simulink model "dinamicaralik"  (R2023b)
settings: Solver=ode45  StartTime=0.0  StopTime=50  FixedStep=0.0001  RelTol=1e-3
InitFcn:
  | Kpz = 0.3 ;
  | KIz = 0;
  | 
  | bh = 0.010290;  % batan hacim m^3
  | m = 10.5     ;  % aracın kütlesi kg
  | g = 9.81     ;  % yer çekimi ivmesi
  | p = 1000     ; % kg / m^3 yogunluk
  | W = m*g      ;  % aracın agırlıgı N
  | B = p*g*bh   ;  % Kaldırma kuvveti  N
  | 
  | xg = 0 ; % rgid body frame e göre ağırlık merkzi kordinatları
  | yg = 0 ;
  | zg = 0.02 ;
  | 
  | Ix = 0.1011 ; % kg *  m ^2
  | Iy = 0.1159 ;
  | Iz = 0.1615 ;
  | 
  | thrustCoefficient = 50/21.5 ;
  | 
  | % Add mass parametreleri
  | Xu_dot = -5.5;   % Surge direction
  | Yv_dot = -12.7;  % Sway direction
  | Zw_dot = -14.57; % Heave direction
  | 
  | Kp_dot = -0.12;  % Roll moment
  | Mq_dot = -0.12;  % Pitch moment
  | Nr_dot = -0.12;  % Yaw moment
  | 
  | % Linear Damping Values (Doğrusal Sönümleme Katsayıları)
  | Xu = -4.03;   % Ns/m
  | Yv = -6.22;   % Ns/m
  | Zw = -5.18;   % Ns/m
  | Kp = -0.07;   % Ns/rad
  | Mq = -0.07;   % Ns/rad
  | Nr = -0.07;   % Ns/rad
  | 
  | % Quadratic Damping Values (Doğrusal Olmayan Sönümleme Katsayıları)
  | Xuu = -18.18;  % Ns^2/m^2
  | Yvv = -21.66;  % Ns^2/m^2
  | Zww = -36.99;  % Ns^2/m^2
  | Kpp = -1.55;   % Ns^2/rad^2
  | Mqq = -1.55;   % Ns^2/rad^2
  | Nrr = -1.55;   % Ns^2/rad^2
undefined symbols (not defined in the file or in its folder): smiData, X, Y, Z
libraries: slpidlib x41, nesl_utility x14, sm_lib x12
(part 7 of 7)

== matlab function dinamicaralik/Subsystem3/CRB/MATLAB Function ==
  data: V input; y output
function y = fcn(V)

u = V(1);
v = V(2);
w = V(3);

p = V(4);
q = V(5);
r = V(6);

Ix = 0.1011 ; % kg *  m ^2 
Iy = 0.1159 ;
Iz = 0.1615 ;

m = 10.5     ;  % aracın kütlesi kg

% Matrisin tanımlanması
CRB = [
        0,     0,     0,        0,   m*w,    0;
        0,     0,     0,     -m*w,     0,    0;
        0,     0,     0,      m*v,  -m*u,    0;
        0,     m*w,  -m*v,    0,     Iz*r,  -Iy*q;
        m*w,  0,    -m*u,   -Iz*r,    0,    Ix*p;
        -m*v,  -m*u,   0,      Iy*q, -Ix*p,   0;
    ];

y= CRB * V ;

== matlab function dinamicaralik/Subsystem3/Damp/MATLAB Function ==
  data: Vw input; y output
function y = fcn(Vw)

u = Vw(1);
v = Vw(2);
w = Vw(3);
p = Vw(4);
q = Vw(5);
r = Vw(6);

% Linear Damping Values (Doğrusal Sönümleme Katsayıları)
Xu = -4.03;   % Ns/m
Yv = -6.22;   % Ns/m
Zw = -5.18;   % Ns/m
Kp = -0.07;   % Ns/rad
Mq = -0.07;   % Ns/rad
Nr = -0.07;   % Ns/rad

% Quadratic Damping Values (Doğrusal Olmayan Sönümleme Katsayıları)
Xuu = -18.18;  % Ns^2/m^2
Yvv = -21.66;  % Ns^2/m^2
Zww = -36.99;  % Ns^2/m^2
Kpp = -1.55;   % Ns^2/rad^2
Mqq = -1.55;   % Ns^2/rad^2
Nrr = -1.55;   % Ns^2/rad^2


D = -[
        Xu + Xuu*abs(u),         0,                 0,                0,                0,                0;
                  0,   Yv + Yvv*abs(v),             0,                0,                0,                0;
                  0,            0,     Zw + Zww*abs(w),             0,                0,                0;
                  0,            0,                 0,   Kp + Kpp*abs(p),             0,                0;
                  0,            0,                 0,                0,   Mq + Mqq*abs(q),             0;
                  0,            0,                 0,                0,                0,   Nr + Nrr*abs(r);
    ];


y = D * Vw ;

== matlab function dinamicaralik/Subsystem3/MA/MATLAB Function ==
  data: accelW input; y output
function y = fcn(accelW)
% Add mass parametreleri
Xu_dot = -5.5;   % Surge direction
Yv_dot = -12.7;  % Sway direction
Zw_dot = -14.57; % Heave direction

Kp_dot = -0.12;  % Roll moment
Mq_dot = -0.12;  % Pitch moment
Nr_dot = -0.12;  % Yaw moment

% MA Matrisinin tanımlanması
MA = -[
        Xu_dot,    0,       0,       0,       0,       0;
        0,       Yv_dot,    0,       0,       0,       0;
        0,         0,     Zw_dot,    0,       0,       0;
        0,         0,       0,     Kp_dot,   0,       0;
        0,         0,       0,       0,     Mq_dot,   0;
        0,         0,       0,       0,       0,     Nr_dot
    ];

y = MA * accelW;

== matlab function dinamicaralik/Subsystem3/inv MA and MRB/MA ve MRB ==
  data: u input; y output
function y = fcn(u)

m = 10.5     ;  % aracın kütlesi kg

xg = 0 ; % rgid body frame e göre ağırlık merkzi kordinatları
yg = 0 ;
zg = 0.02;

Ix = 0.1011 ; % kg *  m ^2 
Iy = 0.1159 ;
Iz = 0.1615 ;


% MRB Matrisinin tanımlanması
MRB = [
        m,    0,    0,    0,   m*zg,  0;
        0,    m,    0, -m*zg,   0,    0;
        0,    0,    m,    0,    0,    0;
        0, -m*zg,   0,   Ix,    0,    0;
       m*zg,  0,    0,    0,   Iy,    0;
        0,    0,    0,    0,    0,   Iz
    ];


Xu_dot = -5.5;   % Surge direction
Yv_dot = -12.7;  % Sway direction
Zw_dot = -14.57; % Heave direction

Kp_dot = -0.12;  % Roll moment
Mq_dot = -0.12;  % Pitch moment
Nr_dot = -0.12;  % Yaw moment

% MA Matrisinin tanımlanması
MA = -[
        Xu_dot,    0,       0,       0,       0,       0;
        0,       Yv_dot,    0,       0,       0,       0;
        0,         0,     Zw_dot,    0,       0,       0;
        0,         0,       0,     Kp_dot,   0,       0;
        0,         0,       0,       0,     Mq_dot,   0;
        0,         0,       0,       0,       0,     Nr_dot
    ];

%inv([m 0 0 0 0 0;0 m 0 0 0 0;0 0 m 0 0 0;0 0 0 Ix 0 0;0 0 0 0 Iy 0;0 0 0 0 0 Iz]+[Xudot 0 0 0 0 0;0 Yvdot 0 0 0 0;0 0 Zwdot 0 0 0;0 0 0 Kpdot 0 0;0 0 0 0 Mqdot 0;0 0 0 0 0 Nrdot])
y = inv(MRB + MA) * u ; % M_product * y = u denkleminden y'i çözer

== matlab function dinamicaralik/Subsystem3/inv MA and MRB/MRB sadece ==
  data: u input; y output
function y = fcn(u)

m = 10.5     ;  % aracın kütlesi kg

xg = 0 ; % rgid body frame e göre ağırlık merkzi kordinatları
yg = 0 ;
zg = 0.02 ;

Ix = 0.1011 ; % kg *  m ^2 
Iy = 0.1159 ;
Iz = 0.1615 ;


% MRB Matrisinin tanımlanması
MRB = [
        m,    0,    0,    0,   m*zg,  0;
        0,    m,    0, -m*zg,   0,    0;
        0,    0,    m,    0,    0,    0;
        0, -m*zg,   0,   Ix,    0,    0;
       m*zg,  0,    0,    0,   Iy,    0;
        0,    0,    0,    0,    0,   Iz
    ];


y = (MRB) \ u ; % M_product * y = u denkleminden y'i çözer

== matlab function dinamicaralik/Subsystem4/MATLAB Function ==
  data: F1 input; thrust1 output
function thrust1 = fcn(F1)

% T1
lx1 = 156 / 1000;  % metre
ly1 = 111 / 1000;  % metre
lz1 = 85 / 1000;   % metre
F1q = pi/4;

Fx = F1 * cos(F1q);
Fy = -F1 * sin(F1q);
Fz = 0;

% Matrisin tanımlanması
forces_and_moments = [
    Fx;                  % Kuvvet: x bileşeni
    Fy;                  % Kuvvet: y bileşeni
    Fz;                  % Kuvvet: z bileşeni
    Fz*ly1 - Fy*lz1;    % Moment: x ekseni etrafında
    Fx*lz1 - Fz*lx1;    % Moment: y ekseni etrafında
    Fy*lx1 - Fx*ly1     % Moment: z ekseni etrafında
];
% Sonuçların görüntülenmesi
%disp('Forces and Moments Matrix:');
%disp(forces_and_moments);

thrust1 = forces_and_moments;

== matlab function dinamicaralik/Subsystem4/MATLAB Function1 ==
  data: F2 input; thrust2 output
function thrust2 = fcn(F2)

% T2
lx2 = 156 / 1000;  % metre
ly2 = -111 / 1000; % metre
lz2 = 85 / 1000;   % metre
F2q = pi/4;

Fx = F2 * cos(F2q);
Fy = F2 * sin(F2q);
Fz = 0;

% Matrisin tanımlanması
forces_and_moments = [
    Fx;                  % Kuvvet: x bileşeni
    Fy;                  % Kuvvet: y bileşeni
    Fz;                  % Kuvvet: z bileşeni
    Fz*ly2 - Fy*lz2;    % Moment: x ekseni etrafında
    Fx*lz2 - Fz*lx2;    % Moment: y ekseni etrafında
    (Fy*lx2 - Fx*ly2)     % Moment: z ekseni etrafında burda liva farklı yapmıs
];
% Sonuçların görüntülenmesi
%disp('Forces and Moments Matrix:');
%disp(forces_and_moments);

thrust2 = forces_and_moments;

== matlab function dinamicaralik/Subsystem4/MATLAB Function10 ==
  data: F3 input; thrust3 output
function thrust3 = fcn(F3)

% T3
lx3 = -156 / 1000; % metre
ly3 = 111 / 1000;  % metre
lz3 = 85 / 1000;   % metre
F3q = pi/4;


Fx = -F3 * cos(F3q);
Fy = -F3 * sin(F3q);
Fz = 0;

% Matrisin tanımlanması
forces_and_moments = [
    Fx;                  % Kuvvet: x bileşeni
    Fy;                  % Kuvvet: y bileşeni
    Fz;                  % Kuvvet: z bileşeni
    Fz*ly3 - Fy*lz3;    % Moment: x ekseni etrafında
    Fx*lz3 - Fz*lx3;    % Moment: y ekseni etrafında
    (Fy*lx3 - Fx*ly3)     % Moment: z ekseni etrafında burda da bi fark var
];
% Sonuçların görüntülenmesi
%disp('Forces and Moments Matrix:');
%disp(forces_and_moments);

thrust3 = forces_and_moments;

== matlab function dinamicaralik/Subsystem4/MATLAB Function11 ==
  data: F4 input; thrust4 output
function thrust4 = fcn(F4)

% T4
lx4 = -156 / 1000; % metre
ly4 = -111 / 1000; % metre
lz4 = 85 / 1000;   % metre
F4q = pi/4;

Fx = -F4 * cos(F4q);
Fy = F4 * sin(F4q);
Fz = 0;

% Matrisin tanımlanması
forces_and_moments = [
    Fx;                  % Kuvvet: x bileşeni
    Fy;                  % Kuvvet: y bileşeni
    Fz;                  % Kuvvet: z bileşeni
    Fz*ly4 - Fy*lz4;    % Moment: x ekseni etrafında
    Fx*lz4 - Fz*lx4;    % Moment: y ekseni etrafında
    (Fy*lx4 - Fx*ly4)     % Moment: z ekseni etrafında bu da farkli
];
% Sonuçların görüntülenmesi
%disp('Forces and Moments Matrix:');
%disp(forces_and_moments);

thrust4 = forces_and_moments;

== matlab function dinamicaralik/Subsystem4/MATLAB Function12 ==
  data: F5 input; thrust5 output
function thrust5 = fcn(F5)

% T5
lx5 = 120 / 1000;  % metre
ly5 = 218 / 1000;  % metre
lz5 = 0 / 1000;    % metre

Fx = 0*F5;
Fy = 0*F5;
Fz = -1*F5;

% Matrisin tanımlanması
forces_and_moments = [
    Fx;                  % Kuvvet: x bileşeni
    Fy;                  % Kuvvet: y bileşeni
    Fz;                  % Kuvvet: z bileşeni
    Fz*ly5 - Fy*lz5;    % Moment: x ekseni etrafında
    Fx*lz5 - Fz*lx5;    % Moment: y ekseni etrafında
    Fy*lx5 - Fx*ly5     % Moment: z ekseni etrafında
];


thrust5 = forces_and_moments;

== matlab function dinamicaralik/Subsystem/Damp/MATLAB Function ==
  data: Vw input; y output
function y = fcn(Vw)

u = Vw(1);
v = Vw(2);
w = Vw(3);
p = Vw(4);
q = Vw(5);
r = Vw(6);

% Linear Damping Values (Doğrusal Sönümleme Katsayıları)
Xu = -4.03;   % Ns/m
Yv = -6.22;   % Ns/m
Zw = -5.18;   % Ns/m
Kp = -0.07;   % Ns/rad
Mq = -0.07;   % Ns/rad
Nr = -0.07;   % Ns/rad

% Quadratic Damping Values (Doğrusal Olmayan Sönümleme Katsayıları)
Xuu = -18.18;  % Ns^2/m^2
Yvv = -21.66;  % Ns^2/m^2
Zww = -36.99;  % Ns^2/m^2
Kpp = -1.55;   % Ns^2/rad^2
Mqq = -1.55;   % Ns^2/rad^2
Nrr = -1.55;   % Ns^2/rad^2


D = -[
        Xu + Xuu*abs(u),         0,                 0,                0,                0,                0;
                  0,   Yv + Yvv*abs(v),             0,                0,                0,                0;
                  0,            0,     Zw + Zww*abs(w),             0,                0,                0;
                  0,            0,                 0,   Kp + Kpp*abs(p),             0,                0;
                  0,            0,                 0,                0,   Mq + Mqq*abs(q),             0;
                  0,            0,                 0,                0,                0,   Nr + Nrr*abs(r);
    ];


y = D * Vw ;

== matlab function dinamicaralik/Subsystem4/MATLAB Function13 ==
  data: F6 input; thrust6 output
function thrust6 = fcn(F6)


% T6
lx6 = 120 / 1000;  % metre
ly6 = -218 / 1000; % metre
lz6 = 0 / 1000;    % metre


Fx = 0*F6;
Fy = 0*F6;
Fz = 1*F6;

% Matrisin tanımlanması
forces_and_moments = [
    Fx;                  % Kuvvet: x bileşeni
    Fy;                  % Kuvvet: y bileşeni
    Fz;                  % Kuvvet: z bileşeni
    Fz*ly6 - Fy*lz6;    % Moment: x ekseni etrafında
    Fx*lz6 - Fz*lx6;    % Moment: y ekseni etrafında
    Fy*lx6 - Fx*ly6     % Moment: z ekseni etrafında
];
% Sonuçların görüntülenmesi
%disp('Forces and Moments Matrix:');
%disp(forces_and_moments);

thrust6 = forces_and_moments;

== matlab function dinamicaralik/Subsystem4/MATLAB Function14 ==
  data: F7 input; thrust7 output
function thrust7 = fcn(F7)

% T7
lx7 = -120 / 1000; % metre
ly7 = 218 / 1000;  % metre
lz7 = 0 / 1000;    % metre

Fx = 0*F7;
Fy = 0*F7;
Fz = 1*F7;

% Matrisin tanımlanması
forces_and_moments = [
    Fx;                  % Kuvvet: x bileşeni
    Fy;                  % Kuvvet: y bileşeni
    Fz;                  % Kuvvet: z bileşeni
    Fz*ly7 - Fy*lz7;    % Moment: x ekseni etrafında
    Fx*lz7 - Fz*lx7;    % Moment: y ekseni etrafında
    Fy*lx7 - Fx*ly7     % Moment: z ekseni etrafında
];
% Sonuçların görüntülenmesi
disp('Forces and Moments Matrix:');
disp(forces_and_moments);

thrust7 = forces_and_moments;

== matlab function dinamicaralik/Subsystem4/MATLAB Function15 ==
  data: F8 input; thrust8 output
function thrust8 = fcn(F8)

% T8
lx8 = -120 / 1000; % metre
ly8 = -218 / 1000; % metre
lz8 = 0 / 1000;    % metre

Fx = 0*F8;
Fy = 0*F8;
Fz = -1*F8;

% Matrisin tanımlanması
forces_and_moments = [
    Fx;                  % Kuvvet: x bileşeni
    Fy;                  % Kuvvet: y bileşeni
    Fz;                  % Kuvvet: z bileşeni
    Fz*ly8 - Fy*lz8;    % Moment: x ekseni etrafında
    Fx*lz8 - Fz*lx8;    % Moment: y ekseni etrafında
    Fy*lx8 - Fx*ly8     % Moment: z ekseni etrafında
];
% Sonuçların görüntülenmesi
disp('Forces and Moments Matrix:');
disp(forces_and_moments);

thrust8 = forces_and_moments;

== matlab function dinamicaralik/Subsystem4/MATLAB Function2 ==
  data: F3 input; thrust3 output
function thrust3 = fcn(F3)

% T3
lx3 = -156 / 1000; % metre
ly3 = 111 / 1000;  % metre
lz3 = 85 / 1000;   % metre
F3q = pi/4;


Fx = -F3 * cos(F3q);
Fy = -F3 * sin(F3q);
Fz = 0;

% Matrisin tanımlanması
forces_and_moments = [
    Fx;                  % Kuvvet: x bileşeni
    Fy;                  % Kuvvet: y bileşeni
    Fz;                  % Kuvvet: z bileşeni
    Fz*ly3 - Fy*lz3;    % Moment: x ekseni etrafında
    Fx*lz3 - Fz*lx3;    % Moment: y ekseni etrafında
    (Fy*lx3 - Fx*ly3)     % Moment: z ekseni etrafında burda da bi fark var
];
% Sonuçların görüntülenmesi
%disp('Forces and Moments Matrix:');
%disp(forces_and_moments);

thrust3 = forces_and_moments;

== matlab function dinamicaralik/Subsystem4/MATLAB Function3 ==
  data: F4 input; thrust4 output
function thrust4 = fcn(F4)

% T4
lx4 = -156 / 1000; % metre
ly4 = -111 / 1000; % metre
lz4 = 85 / 1000;   % metre
F4q = pi/4;

Fx = -F4 * cos(F4q);
Fy = F4 * sin(F4q);
Fz = 0;

% Matrisin tanımlanması
forces_and_moments = [
    Fx;                  % Kuvvet: x bileşeni
    Fy;                  % Kuvvet: y bileşeni
    Fz;                  % Kuvvet: z bileşeni
    Fz*ly4 - Fy*lz4;    % Moment: x ekseni etrafında
    Fx*lz4 - Fz*lx4;    % Moment: y ekseni etrafında
    Fy*lx4 - Fx*ly4     % Moment: z ekseni etrafında bu da farkli
];
% Sonuçların görüntülenmesi
%disp('Forces and Moments Matrix:');
%disp(forces_and_moments);

thrust4 = forces_and_moments;

== matlab function dinamicaralik/Subsystem4/MATLAB Function4 ==
  data: F5 input; thrust5 output
function thrust5 = fcn(F5)

% T5
lx5 = 120 / 1000;  % metre
ly5 = 218 / 1000;  % metre
lz5 = 0 / 1000;    % metre

Fx = 0*F5;
Fy = 0*F5;
Fz = -1*F5;

% Matrisin tanımlanması
forces_and_moments = [
    Fx;                  % Kuvvet: x bileşeni
    Fy;                  % Kuvvet: y bileşeni
    Fz;                  % Kuvvet: z bileşeni
    Fz*ly5 - Fy*lz5;    % Moment: x ekseni etrafında
    Fx*lz5 - Fz*lx5;    % Moment: y ekseni etrafında
    Fy*lx5 - Fx*ly5     % Moment: z ekseni etrafında
];


thrust5 = forces_and_moments;

== matlab function dinamicaralik/Subsystem4/MATLAB Function5 ==
  data: F6 input; thrust6 output
function thrust6 = fcn(F6)


% T6
lx6 = 120 / 1000;  % metre
ly6 = -218 / 1000; % metre
lz6 = 0 / 1000;    % metre


Fx = 0*F6;
Fy = 0*F6;
Fz = 1*F6;

% Matrisin tanımlanması
forces_and_moments = [
    Fx;                  % Kuvvet: x bileşeni
    Fy;                  % Kuvvet: y bileşeni
    Fz;                  % Kuvvet: z bileşeni
    Fz*ly6 - Fy*lz6;    % Moment: x ekseni etrafında
    Fx*lz6 - Fz*lx6;    % Moment: y ekseni etrafında
    Fy*lx6 - Fx*ly6     % Moment: z ekseni etrafında
];
% Sonuçların görüntülenmesi
%disp('Forces and Moments Matrix:');
%disp(forces_and_moments);

thrust6 = forces_and_moments;

== matlab function dinamicaralik/Subsystem4/MATLAB Function6 ==
  data: F7 input; thrust7 output
function thrust7 = fcn(F7)

% T7
lx7 = -120 / 1000; % metre
ly7 = 218 / 1000;  % metre
lz7 = 0 / 1000;    % metre

Fx = 0*F7;
Fy = 0*F7;
Fz = 1*F7;

% Matrisin tanımlanması
forces_and_moments = [
    Fx;                  % Kuvvet: x bileşeni
    Fy;                  % Kuvvet: y bileşeni
    Fz;                  % Kuvvet: z bileşeni
    Fz*ly7 - Fy*lz7;    % Moment: x ekseni etrafında
    Fx*lz7 - Fz*lx7;    % Moment: y ekseni etrafında
    Fy*lx7 - Fx*ly7     % Moment: z ekseni etrafında
];
% Sonuçların görüntülenmesi
disp('Forces and Moments Matrix:');
disp(forces_and_moments);

thrust7 = forces_and_moments;

== matlab function dinamicaralik/Subsystem4/MATLAB Function7 ==
  data: F8 input; thrust8 output
function thrust8 = fcn(F8)

% T8
lx8 = -120 / 1000; % metre
ly8 = -218 / 1000; % metre
lz8 = 0 / 1000;    % metre

Fx = 0*F8;
Fy = 0*F8;
Fz = -1*F8;

% Matrisin tanımlanması
forces_and_moments = [
    Fx;                  % Kuvvet: x bileşeni
    Fy;                  % Kuvvet: y bileşeni
    Fz;                  % Kuvvet: z bileşeni
    Fz*ly8 - Fy*lz8;    % Moment: x ekseni etrafında
    Fx*lz8 - Fz*lx8;    % Moment: y ekseni etrafında
    Fy*lx8 - Fx*ly8     % Moment: z ekseni etrafında
];
% Sonuçların görüntülenmesi
disp('Forces and Moments Matrix:');
disp(forces_and_moments);

thrust8 = forces_and_moments;

== matlab function dinamicaralik/Subsystem4/MATLAB Function8 ==
  data: F1 input; thrust1 output
function thrust1 = fcn(F1)

% T1
lx1 = 156 / 1000;  % metre
ly1 = 111 / 1000;  % metre
lz1 = 85 / 1000;   % metre
F1q = pi/4;

Fx = F1 * cos(F1q);
Fy = -F1 * sin(F1q);
Fz = 0;

% Matrisin tanımlanması
forces_and_moments = [
    Fx;                  % Kuvvet: x bileşeni
    Fy;                  % Kuvvet: y bileşeni
    Fz;                  % Kuvvet: z bileşeni
    Fz*ly1 - Fy*lz1;    % Moment: x ekseni etrafında
    Fx*lz1 - Fz*lx1;    % Moment: y ekseni etrafında
    Fy*lx1 - Fx*ly1     % Moment: z ekseni etrafında
];
% Sonuçların görüntülenmesi
%disp('Forces and Moments Matrix:');
%disp(forces_and_moments);

thrust1 = forces_and_moments;

== matlab function dinamicaralik/Subsystem1/MATLAB Function ==
  data: F1 input; thrust1 output
function thrust1 = fcn(F1)

% T1
lx1 = 156 / 1000;  % metre
ly1 = 111 / 1000;  % metre
lz1 = 85 / 1000;   % metre
F1q = pi/4;

Fx = F1 * cos(F1q);
Fy = -F1 * sin(F1q);
Fz = 0;

% Matrisin tanımlanması
forces_and_moments = [
    Fx;                  % Kuvvet: x bileşeni
    Fy;                  % Kuvvet: y bileşeni
    Fz;                  % Kuvvet: z bileşeni
    Fz*ly1 - Fy*lz1;    % Moment: x ekseni etrafında
    Fx*lz1 - Fz*lx1;    % Moment: y ekseni etrafında
    Fy*lx1 - Fx*ly1     % Moment: z ekseni etrafında
];
% Sonuçların görüntülenmesi
%disp('Forces and Moments Matrix:');
%disp(forces_and_moments);

thrust1 = forces_and_moments;

== matlab function dinamicaralik/Subsystem4/MATLAB Function9 ==
  data: F2 input; thrust2 output
function thrust2 = fcn(F2)

% T2
lx2 = 156 / 1000;  % metre
ly2 = -111 / 1000; % metre
lz2 = 85 / 1000;   % metre
F2q = pi/4;

Fx = F2 * cos(F2q);
Fy = F2 * sin(F2q);
Fz = 0;

% Matrisin tanımlanması
forces_and_moments = [
    Fx;                  % Kuvvet: x bileşeni
    Fy;                  % Kuvvet: y bileşeni
    Fz;                  % Kuvvet: z bileşeni
    Fz*ly2 - Fy*lz2;    % Moment: x ekseni etrafında
    Fx*lz2 - Fz*lx2;    % Moment: y ekseni etrafında
    (Fy*lx2 - Fx*ly2)     % Moment: z ekseni etrafında burda liva farklı yapmıs
];
% Sonuçların görüntülenmesi
%disp('Forces and Moments Matrix:');
%disp(forces_and_moments);

thrust2 = forces_and_moments;

== matlab function dinamicaralik/pwm to fource1/MATLAB Function1 ==
  data: u input; y output
function y = Normalize(u)
y = (u-1500)*150/400;

== matlab function dinamicaralik/pwm to fource1/MATLAB Function2 ==
  data: u input; y output
function y = Normalize(u)
y = (u-1500)*150/400;

== matlab function dinamicaralik/pwm to fource1/MATLAB Function3 ==
  data: u input; y output
function y = Normalize(u)
y = (u-1500)*150/400;

== matlab function dinamicaralik/pwm to fource1/MATLAB Function4 ==
  data: u input; y output
function y = Normalize(u)
y = (u-1500)*150/400;

== matlab function dinamicaralik/pwm to fource1/MATLAB Function5 ==
  data: u input; y output
function y = Normalize(u)
y = (u-1500)*150/400;

== matlab function dinamicaralik/pwm to fource1/MATLAB Function6 ==
  data: u input; y output
function y = Normalize(u)
y = (u-1500)*150/400;

== matlab function dinamicaralik/pwm to fource1/MATLAB Function7 ==
  data: u input; y output
function y = Normalize(u)
y = (u-1500)*150/400;

== matlab function dinamicaralik/pwm to fource1/MATLAB Function8 ==
  data: u input; y output
function y = Normalize(u)
y = (u-1500)*150/400;

== matlab function dinamicaralik/Invers Kinematic/euler transform ==
  data: NEDpos input; posB output
function posB = fcn(NEDpos)

phi = -pi;

theta = 0;

psi = 0;

Rbn = [
    cos(psi)*cos(theta), -sin(psi)*cos(phi) + cos(psi)*sin(theta)*sin(phi),  sin(psi)*sin(phi) + cos(psi)*cos(phi)*sin(theta);
    sin(psi)*cos(theta),  cos(psi)*cos(phi) + sin(psi)*sin(theta)*sin(phi), -cos(psi)*sin(phi) + sin(psi)*cos(phi)*sin(theta);
   -sin(theta),          cos(theta)*sin(phi),                              cos(theta)*cos(phi)
];


Ttheta = [
    1, sin(phi)*tan(theta), cos(phi)*tan(theta);
    0, cos(phi),           -sin(phi);
    0, sin(phi)/cos(theta), cos(phi)/cos(theta)
];

% 0_3x3 sıfır matrisi
Zero3x3 = zeros(3);

% Jacobian matrisi J_Theta(eta)
JTheta = [
    Rbn,      Zero3x3;
    Zero3x3,  Ttheta
];


posB = JTheta' * NEDpos ;

== matlab function dinamicaralik/Subsystem1/MATLAB Function1 ==
  data: F2 input; thrust2 output
function thrust2 = fcn(F2)

% T2
lx2 = 156 / 1000;  % metre
ly2 = -111 / 1000; % metre
lz2 = 85 / 1000;   % metre
F2q = pi/4;

Fx = F2 * cos(F2q);
Fy = F2 * sin(F2q);
Fz = 0;

% Matrisin tanımlanması
forces_and_moments = [
    Fx;                  % Kuvvet: x bileşeni
    Fy;                  % Kuvvet: y bileşeni
    Fz;                  % Kuvvet: z bileşeni
    Fz*ly2 - Fy*lz2;    % Moment: x ekseni etrafında
    Fx*lz2 - Fz*lx2;    % Moment: y ekseni etrafında
    (Fy*lx2 - Fx*ly2)     % Moment: z ekseni etrafında burda liva farklı yapmıs
];
% Sonuçların görüntülenmesi
%disp('Forces and Moments Matrix:');
%disp(forces_and_moments);

thrust2 = forces_and_moments;

== matlab function dinamicaralik/Subsystem1/MATLAB Function2 ==
  data: F3 input; thrust3 output
function thrust3 = fcn(F3)

% T3
lx3 = -156 / 1000; % metre
ly3 = 111 / 1000;  % metre
lz3 = 85 / 1000;   % metre
F3q = pi/4;


Fx = -F3 * cos(F3q);
Fy = -F3 * sin(F3q);
Fz = 0;

% Matrisin tanımlanması
forces_and_moments = [
    Fx;                  % Kuvvet: x bileşeni
    Fy;                  % Kuvvet: y bileşeni
    Fz;                  % Kuvvet: z bileşeni
    Fz*ly3 - Fy*lz3;    % Moment: x ekseni etrafında
    Fx*lz3 - Fz*lx3;    % Moment: y ekseni etrafında
    (Fy*lx3 - Fx*ly3)     % Moment: z ekseni etrafında burda da bi fark var
];
% Sonuçların görüntülenmesi
%disp('Forces and Moments Matrix:');
%disp(forces_and_moments);

thrust3 = forces_and_moments;

== matlab function dinamicaralik/Subsystem1/MATLAB Function3 ==
  data: F4 input; thrust4 output
function thrust4 = fcn(F4)

% T4
lx4 = -156 / 1000; % metre
ly4 = -111 / 1000; % metre
lz4 = 85 / 1000;   % metre
F4q = pi/4;

Fx = -F4 * cos(F4q);
Fy = F4 * sin(F4q);
Fz = 0;

% Matrisin tanımlanması
forces_and_moments = [
    Fx;                  % Kuvvet: x bileşeni
    Fy;                  % Kuvvet: y bileşeni
    Fz;                  % Kuvvet: z bileşeni
    Fz*ly4 - Fy*lz4;    % Moment: x ekseni etrafında
    Fx*lz4 - Fz*lx4;    % Moment: y ekseni etrafında
    Fy*lx4 - Fx*ly4     % Moment: z ekseni etrafında bu da farkli
];
% Sonuçların görüntülenmesi
%disp('Forces and Moments Matrix:');
%disp(forces_and_moments);

thrust4 = forces_and_moments;

== matlab function dinamicaralik/Subsystem1/MATLAB Function4 ==
  data: F5 input; thrust5 output
function thrust5 = fcn(F5)

% T5
lx5 = 120 / 1000;  % metre
ly5 = 218 / 1000;  % metre
lz5 = 0 / 1000;    % metre

Fx = 0*F5;
Fy = 0*F5;
Fz = -1*F5;

% Matrisin tanımlanması
forces_and_moments = [
    Fx;                  % Kuvvet: x bileşeni
    Fy;                  % Kuvvet: y bileşeni
    Fz;                  % Kuvvet: z bileşeni
    Fz*ly5 - Fy*lz5;    % Moment: x ekseni etrafında
    Fx*lz5 - Fz*lx5;    % Moment: y ekseni etrafında
    Fy*lx5 - Fx*ly5     % Moment: z ekseni etrafında
];


thrust5 = forces_and_moments;

== matlab function dinamicaralik/Subsystem1/MATLAB Function5 ==
  data: F6 input; thrust6 output
function thrust6 = fcn(F6)


% T6
lx6 = 120 / 1000;  % metre
ly6 = -218 / 1000; % metre
lz6 = 0 / 1000;    % metre


Fx = 0*F6;
Fy = 0*F6;
Fz = 1*F6;

% Matrisin tanımlanması
forces_and_moments = [
    Fx;                  % Kuvvet: x bileşeni
    Fy;                  % Kuvvet: y bileşeni
    Fz;                  % Kuvvet: z bileşeni
    Fz*ly6 - Fy*lz6;    % Moment: x ekseni etrafında
    Fx*lz6 - Fz*lx6;    % Moment: y ekseni etrafında
    Fy*lx6 - Fx*ly6     % Moment: z ekseni etrafında
];
% Sonuçların görüntülenmesi
%disp('Forces and Moments Matrix:');
%disp(forces_and_moments);

thrust6 = forces_and_moments;

== matlab function dinamicaralik/Subsystem1/MATLAB Function6 ==
  data: F7 input; thrust7 output
function thrust7 = fcn(F7)

% T7
lx7 = -120 / 1000; % metre
ly7 = 218 / 1000;  % metre
lz7 = 0 / 1000;    % metre

Fx = 0*F7;
Fy = 0*F7;
Fz = 1*F7;

% Matrisin tanımlanması
forces_and_moments = [
    Fx;                  % Kuvvet: x bileşeni
    Fy;                  % Kuvvet: y bileşeni
    Fz;                  % Kuvvet: z bileşeni
    Fz*ly7 - Fy*lz7;    % Moment: x ekseni etrafında
    Fx*lz7 - Fz*lx7;    % Moment: y ekseni etrafında
    Fy*lx7 - Fx*ly7     % Moment: z ekseni etrafında
];
% Sonuçların görüntülenmesi
disp('Forces and Moments Matrix:');
disp(forces_and_moments);

thrust7 = forces_and_moments;

== matlab function dinamicaralik/Subsystem1/MATLAB Function7 ==
  data: F8 input; thrust8 output
function thrust8 = fcn(F8)

% T8
lx8 = -120 / 1000; % metre
ly8 = -218 / 1000; % metre
lz8 = 0 / 1000;    % metre

Fx = 0*F8;
Fy = 0*F8;
Fz = -1*F8;

% Matrisin tanımlanması
forces_and_moments = [
    Fx;                  % Kuvvet: x bileşeni
    Fy;                  % Kuvvet: y bileşeni
    Fz;                  % Kuvvet: z bileşeni
    Fz*ly8 - Fy*lz8;    % Moment: x ekseni etrafında
    Fx*lz8 - Fz*lx8;    % Moment: y ekseni etrafında
    Fy*lx8 - Fx*ly8     % Moment: z ekseni etrafında
];
% Sonuçların görüntülenmesi
disp('Forces and Moments Matrix:');
disp(forces_and_moments);

thrust8 = forces_and_moments;

== matlab function dinamicaralik/pwm to fource/MATLAB Function8 ==
  data: u input; y output
function y = Normalize(u)
y = (u-1500)*150/400;
